simulink library "FriedrichLibrary"  (R2015b)
settings: Solver=ode45  SolverMode=SingleTasking  StartTime=0.0  StopTime=10.0  RelTol=1e-3
values from neighbouring files (symbols this model uses):
  ControlSampleTime = 1/8000    (= 0.000125)    [initTPHardware.m]
  Ts = ControlSampleTime    [Sim_TP3_VSM_init.m]
undefined symbols (not defined in the file or in its folder): init_out
undefined symbols (not defined in the file): CC1, PLL
libraries: FriedrichLibrary x29, simulink x6, powerlib_meascontrol x1
settings Model: Creator=fwelck  LastModifiedBy=fwelck
settings DataIOCC: SaveFormat=Array
settings OptimizationCC: BlockReduction=off  BooleanDataType=off
settings DebuggingCC: SaveWithParameterizedLinksMsg=none  UnderspecifiedInitializationDetection=Classic  MergeDetectMultiDrivingBlocksExec=none  SignalResolutionControl=TryResolveAllWithWarning  StrictBusMsg=Warning
settings HardwareCC: ProdBitPerPointer=32  ProdLargestAtomicFloat=None  ProdIntDivRoundTo=Undefined  ProdEndianess=Unspecified  ProdWordSize=32  ProdHWDeviceType=32-bit Generic  TargetUnknown=on
settings GRTTargetCC: GeneratePreprocessorConditionals=Disable all
settings ConfigComp: CovModelRefEnable=Off  CovSFcnEnable=off

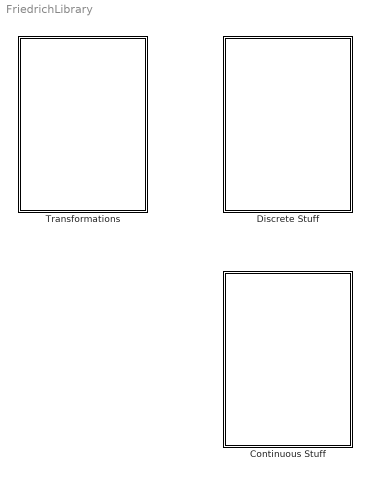
== system FriedrichLibrary ==
  Continuous Stuff : Subsystem
  Discrete Stuff : Subsystem
  Transformations : Subsystem

== system FriedrichLibrary/Continuous Stuff ==
  G.4 First order filter with initial state : Subsystem  mask{T=0.1, init_out=0}
      mask prompts: T "Time constant [s]"; init_out "Initial State"
      mask Display:
      | text(0.5,0.5,'1','HorizontalAlignment','center','VerticalAlignment','Bottom')
      | text(0.5,0.5,['1 + s*' get_param(gcb,'T')],'HorizontalAlignment','center','VerticalAlignment','Top')
      | plot([0.3 0.7],[0.5 0.5])

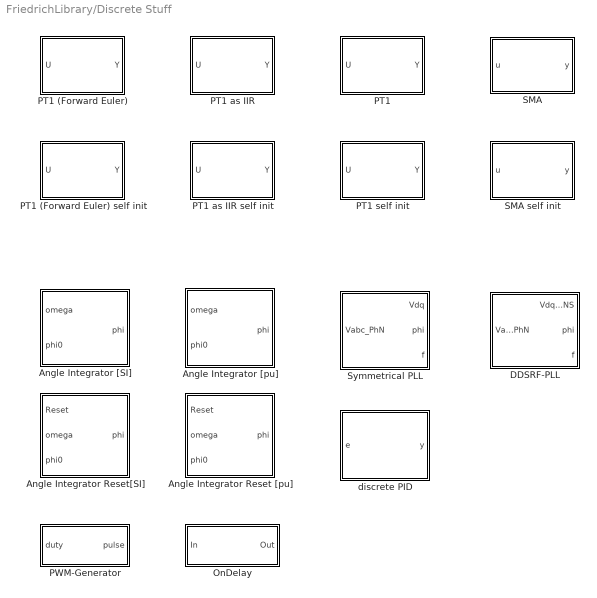
== system FriedrichLibrary/Discrete Stuff ==
  Angle Integrator Reset [pu] : Subsystem  mask{Ts=Ts}
      mask prompts: Ts "SampleTime"
      mask DialogControl DescTextVar Prompt: Discrete Integrator with wrap around at -0.5 and 0.5
  Angle Integrator Reset[SI] : Subsystem  mask{Ts=Ts}
      mask prompts: Ts "SampleTime"
      mask DialogControl DescTextVar Prompt: Discrete Integrator for omega, resetting every 2*pi.
  Angle Integrator [SI] : Subsystem  mask{Ts=Ts}
      mask prompts: Ts "SampleTime"
      mask DialogControl DescTextVar Prompt: Discrete Integrator for omega, resetting every 2*pi.
  Angle Integrator [pu] : Subsystem  mask{Ts=Ts}
      mask prompts: Ts "SampleTime"
      mask DialogControl DescTextVar Prompt: Discrete Integrator with wrap around at -0.5 and 0.5
  DDSRF-PLL : Subsystem  mask{Kp_PLL=PLL.kp, Ki_PLL=PLL.ki, Kd_PLL=0, Tpt1=0.005, Ts=ControlSampleTime}
      mask prompts: Kp_PLL "Proportional Gain PLL"; Ki_PLL "Integral Gain PLL"; Kd_PLL "Differential Gain PLL"; Tpt1 "PT1 Settling Time"; Ts "SampleTime"
      mask DialogControl DescTextVar Prompt: Discrete implementation of a double decoupled sychronous reference frame phase locked loop.
  OnDelay : Subsystem  mask{T_on=2e-6}
      mask prompts: T_on "On Delay Time"
  PT1 : Subsystem  mask{K=1, tau=0.02, Init=0, T=ControlSampleTime}
      mask prompts: K "Gain"; tau "Settling time"; Init "Initial input"; T "Sample time"
      mask DialogControl DescTextVar Prompt: Simple discrete PT1
      mask Display:
      | text(0.5,0.5,get_param(gcb,'K'),'HorizontalAlignment','center','VerticalAlignment','Bottom')
      | text(0.5,0.5,['1 + s*' get_param(gcb,'tau')],'HorizontalAlignment','center','VerticalAlignment','Top')
      | plot([0.3 0.7],[0.5 0.5])
  PT1 self init : Subsystem  mask{K=1, tau=0.02, T=0.001}
      mask prompts: K "Gain"; tau "Settling time"; T "Sample time"
      mask DialogControl DescTextVar Prompt: Simple discrete PT1
      mask Display:
      | text(0.5,0.5,get_param(gcb,'K'),'HorizontalAlignment','center','VerticalAlignment','Bottom')
      | text(0.5,0.5,['1 + s*' get_param(gcb,'tau')],'HorizontalAlignment','center','VerticalAlignment','Top')
      | plot([0.3 0.7],[0.5 0.5])
  PT1 (Forward Euler) : Subsystem  mask{K=1, tau=0.1, Init=0, T=0.001}
      mask prompts: K "Gain"; tau "Settling time [s]"; Init "Initial input"; T "Sample time [s]"
      mask DialogControl DescTextVar Prompt: Forward Euler discretization of a PT1 filter.
      mask Display:
      | text(0.5,0.5,get_param(gcb,'K'),'HorizontalAlignment','center','VerticalAlignment','Bottom')
      | text(0.5,0.5,['1 + s*' get_param(gcb,'tau')],'HorizontalAlignment','center','VerticalAlignment','Top')
      | plot([0.3 0.7],[0.5 0.5])
  PT1 (Forward Euler) self init : Subsystem  mask{K=1, tau=0.1, T=0.001}
      mask prompts: K "Gain"; tau "Settling time [s]"; T "Sample time [s]"
      mask DialogControl DescTextVar Prompt: Forward Euler discretization of a PT1 filter.
      mask Display:
      | text(0.5,0.5,get_param(gcb,'K'),'HorizontalAlignment','center','VerticalAlignment','Bottom')
      | text(0.5,0.5,['1 + s*' get_param(gcb,'tau')],'HorizontalAlignment','center','VerticalAlignment','Top')
      | plot([0.3 0.7],[0.5 0.5])
  PT1 as IIR : Subsystem  mask{K=1, tau=0.02, Init=0, T=ControlSampleTime}
      mask prompts: K "Gain"; tau "Settling time"; Init "Initial input"; T "Sample time"
      mask DialogControl DescTextVar Prompt: IIR form of a PT1 filter
      mask Display:
      | text(0.5,0.5,get_param(gcb,'K'),'HorizontalAlignment','center','VerticalAlignment','Bottom')
      | text(0.5,0.5,['1 + s*' get_param(gcb,'tau')],'HorizontalAlignment','center','VerticalAlignment','Top')
      | plot([0.3 0.7],[0.5 0.5])
  PT1 as IIR self init : Subsystem  mask{K=1, tau=0.02, T=0.001}
      mask prompts: K "Gain"; tau "Settling time"; T "Sample time"
      mask DialogControl DescTextVar Prompt: IIR form of a PT1 filter
      mask Display:
      | text(0.5,0.5,get_param(gcb,'K'),'HorizontalAlignment','center','VerticalAlignment','Bottom')
      | text(0.5,0.5,['1 + s*' get_param(gcb,'tau')],'HorizontalAlignment','center','VerticalAlignment','Top')
      | plot([0.3 0.7],[0.5 0.5])
  PWM-Generator : Subsystem  mask{f_triangle=8000}
      mask prompts: f_triangle "Carrier Frequency"
  SMA : Subsystem  mask{n_samples=3, init_out=0}
      mask prompts: n_samples "Number of samples to average over"; init_out "Initial state"
      mask DialogControl DescTextVar Prompt: Cycle buffer implementation of a simple moving average with initialization. Performs a lot faster than an FIR implementation for averages of 3 samples or more.
  SMA self init : Subsystem  mask{n_samples=3}
      mask prompts: n_samples "Number of samples to average over"
      mask DialogControl DescTextVar Prompt: Cycle buffer implementation of a simple moving average. Performs a lot faster than an FIR implementation for averages of 3 samples or more. Initializes with first input sample.
  Symmetrical PLL : Subsystem  mask{Kp_PLL=CC1.PLL.kp, Ki_PLL=CC1.PLL.ki, Kd_PLL=0, Ts=ControlSampleTime}
      mask prompts: Kp_PLL "Proportional Gain PLL"; Ki_PLL "Integral Gain PLL"; Kd_PLL "Differential Gain PLL"; Ts "SampleTime"
      mask DialogControl DescTextVar Prompt: Discrete implementation of a synchronous reference phase locked loop.
  discrete PID : Subsystem  mask{Kp=1, Ki=2, Kd=3, Ts=ControlSampleTime, x_init=0}
      mask prompts: Kp "Proportional Gain"; Ki "Integral Gain"; Kd "Differential Gain"; Ts "SampleTime"; x_init "Initial Condition"

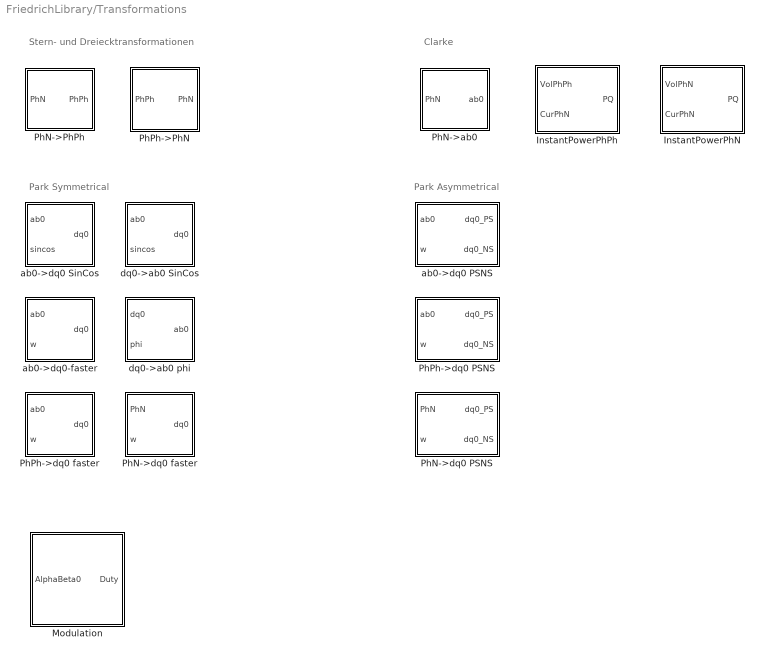
== system FriedrichLibrary/Transformations ==
  note: Park Symmetrical
  note: Park Asymmetrical
  note: Clarke
  note: Stern- und Dreiecktransformationen
  InstantPowerPhN : Subsystem
  InstantPowerPhPh : Subsystem
  Modulation : Subsystem  mask{Method=Sine Modulation, Ts=0}
      mask prompts: Method "Modulation Technique"; Ts "SampleTime"
      mask TypeOptions Method: Standard SpaceVectorModulation | U0N Space Vector Modulation | U7N Space Vector Modulation | Sine Modulation | SineWithThird Modulation
      mask DialogControl DescTextVar Prompt: Performs AlphaBeta0 to ABC conversion via different Modulation Techniques
      mask Display:
      | plot(0,-1,1,1)
      | % Create three 120° shifted sine (3x72)
      | angles = [0:5:360; 120:5:480; 240:5:600]';
      | sine = sind(angles);
      | % Get Maximum and Minimum of all three sine waves
      | Maxi = max(sine,[],2);
      | Mini = min(sine,[],2);
      | % Make them (3x73)
      | Maxi = repmat(Maxi,[1 3]);
      | Mini = repmat(Mini,[1 3]);
      | 
      | switch Method
      |     case 1
      |         plot(angles(:,[1 1 1])/360,sine-(Maxi+Mini)/2);
      |     case 2
      |         plot(angles(:,[1 1 1])/360,sine-Mini-1);
      |     case 3
      |         plot(angles(:,[1 1 1])/360,sine-Maxi+1);
      |     case 4
      |         plot(angles(:,[1 1 1])/360,sine);
      |     case 5
      |         plot(angles(:,[1 1 1])/360,sine-repmat(prod(sine,2)/3*2,[1 3]));
      | end
      | text(0,0,' \alpha\beta0','texmode','on')
      | text(1,0,'duty ','HorizontalAlignment','Right')
  PhN->PhPh : Subsystem
      mask Display:
      | plot([0 1], [0,1])
      | plot([0.1 0.25 0.4 0.25 0.25], [0.5 0.6 0.5 0.6 0.8]) % Stern
      | plot([0.6 0.9 0.75 0.6], [0.2 0.2 0.5 0.2])           % Dreieck
      | text(0.05,1,'PhN','VerticalAlignment','Top')
      | text(1, 0,'PhPh','VerticalAlignment','Bottom','HorizontalAlignment','Right')
  PhN->ab0 : Subsystem
      mask Display:
      | plot([0 1], [0,1])
      | plot([0.1 0.25 0.4 0.25 0.25], [0.5 0.6 0.5 0.6 0.8]) % Stern
      | text(0.05,1,'PhN','VerticalAlignment','Top')
      | text(0.55, 0.3,'\alpha\beta0','texmode','on')
  PhN->dq0 PSNS : Subsystem
      mask Display:
      | plot(0,0,1,1)
      | text(0.05,0.75,'PhN')
      | text(1, 0.75,'dq0_PS','HorizontalAlignment','right')
      | text(1, 0.25,'dq0_NS','HorizontalAlignment','right')
      | text(0.05,0.3,'\phi','texmode','on')
  PhN->dq0 faster : Subsystem
      mask Display:
      | plot([0 1], [0,1])
      | plot([0.1 0.25 0.4 0.25 0.25], [0.5 0.6 0.5 0.6 0.8]) % Stern
      | text(0.05,1,'PhN','VerticalAlignment','Top')
      | text(1, 0.5,'dq0','HorizontalAlignment','right')
      | text(0.05,0.3,'\phi','texmode','on')
  PhPh->PhN : Subsystem
      mask Display:
      | plot([0 1], [0,1])
      | plot([0.6 0.75 0.9 0.75 0.75], [0.2 0.3 0.2 0.3 0.5]) % Stern
      | plot([0.1 0.4 0.25 0.1], [0.5 0.5 0.8 0.5])           % Dreieck
      | text(0.05,1,'PhPh','VerticalAlignment','Top')
      | text(1, 0,'PhN','VerticalAlignment','Bottom','HorizontalAlignment','Right')
  PhPh->dq0 PSNS : Subsystem  mask{Tpt1=0}
      mask prompts: Tpt1 "PT1 Settling Time"
      mask Display:
      | plot(0,0,1,1)
      | text(0.05,0.75,'PhPh')
      | text(1, 0.75,'dq0_PS','HorizontalAlignment','right')
      | text(1, 0.25,'dq0_NS','HorizontalAlignment','right')
      | text(0.05,0.3,'\phi','texmode','on')
  PhPh->dq0 faster : Subsystem
      mask Display:
      | plot([0 1], [0,1])
      | plot([0.1 0.4 0.25 0.1], [0.5 0.5 0.8 0.5])           % Dreieck
      | text(0.05,1,'PhPh','VerticalAlignment','Top')
      | text(1, 0.5,'dq0','HorizontalAlignment','right')
      | text(0.05,0.3,'\phi','texmode','on')
  ab0->dq0 PSNS : Subsystem  mask{T1=0.0045}
      mask prompts: T1 "PT1 Settling Time"
      mask Display:
      | plot(0,0,1,1)
      | text(0.05,0.8,'\alpha\beta0','texmode','on')
      | text(1, 0.75,'dq0_PS','HorizontalAlignment','right')
      | text(1, 0.25,'dq0_NS','HorizontalAlignment','right')
      | text(0.05,0.3,'\phi','texmode','on')
  ab0->dq0 SinCos : Subsystem
      mask Display:
      | plot(0,0,1,1)
      | text(0.05,0.8,'\alpha\beta0','texmode','on')
      | text(1,0.5,'dq0','horizontalalignment','right')
      | text(0.05,0.3,'sincos','texmode','on')
  ab0->dq0-faster : Subsystem
      mask Display:
      | plot([0 1], [0,1])
      | text(0.05,0.8,'\alpha\beta0','texmode','on')
      | text(1, 0.5,'dq0','HorizontalAlignment','right')
      | text(0.05,0.3,'\phi','texmode','on')
  dq0->ab0 SinCos : Subsystem
      mask Display:
      | plot(0,0,1,1)
      | text(0.05,0.8,'dq0')
      | text(1,0.5,'\alpha\beta0','texmode','on','horizontalalignment','right')
      | text(0.05,0.3,'sincos','texmode','on')
  dq0->ab0 phi : Subsystem
      mask Display:
      | plot([0 1], [0,1])
      | text(0.05,0.8,'dq0','texmode','on')
      | text(1, 0.5,'\alpha\beta0','HorizontalAlignment','right','texmode','on')
      | text(0.05,0.3,'\phi','texmode','on')

== system FriedrichLibrary/Continuous Stuff/G.4 First order filter with initial state ==
  x : Inport
  Gain : Gain  Gain=1/T
  Integrator Limited : Integrator  InitialCondition=init_out
  Sum : Sum  Inputs=-+|
  y : Outport
  wires:
  Sum/1 -> Gain/1
  x/1 -> Sum/2
  Gain/1 -> Integrator Limited/1
  Integrator Limited/1 -> Sum/1, y/1

== system FriedrichLibrary/Discrete Stuff/Angle Integrator Reset [pu] ==
  Reset : Inport
  omega : Inport  Port=2
  phi0 : Inport  Port=3
  Bias : Bias  Bias=-1
  Bias1 : Bias  Bias=1
  Delay : Delay  DelayLength=1  InitialConditionSource=Input port  ExternalReset=Rising  SampleTime=Ts
      settings: InputPortMap=u0,r5,p4
  Gain3 : Gain  Gain=Ts
  Sum : Sum  Inputs=|++
  Switch : Switch  Criteria=u2 > Threshold  Threshold=0.5
  Switch1 : Switch  Criteria=u2 > Threshold  Threshold=-0.5
  phi : Outport
  wires:
  phi0/1 -> Delay/3
  Delay/1 -> Sum/2, phi/1
  Switch1/1 -> Delay/1
  Bias1/1 -> Switch1/3
  Switch/1 -> Bias1/1, Switch1/2, Switch1/1
  omega/1 -> Gain3/1
  Gain3/1 -> Sum/1
  Bias/1 -> Switch/1
  Sum/1 -> Switch/3, Switch/2, Bias/1
  Reset/1 -> Delay/2

== system FriedrichLibrary/Discrete Stuff/Angle Integrator Reset[SI] ==
  Reset : Inport
  omega : Inport  Port=2
  phi0 : Inport  Port=3
  Bias : Bias  Bias=-2*pi
  Bias1 : Bias  Bias=2*pi
  Delay : Delay  DelayLength=1  InitialConditionSource=Input port  ExternalReset=Rising  SampleTime=Ts
      settings: InputPortMap=u0,r5,p4
  Gain3 : Gain  Gain=Ts
  Sum : Sum  Inputs=|++
  Switch : Switch  Criteria=u2 > Threshold  Threshold=pi
  Switch1 : Switch  Threshold=-pi
  phi : Outport
  wires:
  Reset/1 -> Delay/2
  phi0/1 -> Delay/3
  omega/1 -> Gain3/1
  Gain3/1 -> Sum/1
  Bias/1 -> Switch/1
  Sum/1 -> Switch/3, Switch/2, Bias/1
  Delay/1 -> phi/1, Sum/2
  Switch/1 -> Switch1/1, Bias1/1, Switch1/2
  Bias1/1 -> Switch1/3
  Switch1/1 -> Delay/1

== system FriedrichLibrary/Discrete Stuff/Angle Integrator [SI] ==
  omega : Inport
  phi0 : Inport  Port=2
  Bias : Bias  Bias=-2*pi
  Bias1 : Bias  Bias=2*pi
  Delay : Delay  DelayLength=1  InitialConditionSource=Input port  SampleTime=Ts
      settings: InputPortMap=u0,p4
  Gain3 : Gain  Gain=Ts
  Sum : Sum  Inputs=|++
  Switch : Switch  Criteria=u2 > Threshold  Threshold=pi
  Switch1 : Switch  Threshold=-pi
  phi : Outport
  wires:
  phi0/1 -> Delay/2
  omega/1 -> Gain3/1
  Gain3/1 -> Sum/1
  Bias/1 -> Switch/1
  Sum/1 -> Switch/3, Switch/2, Bias/1
  Delay/1 -> Sum/2, phi/1
  Switch/1 -> Switch1/1, Bias1/1, Switch1/2
  Bias1/1 -> Switch1/3
  Switch1/1 -> Delay/1

== system FriedrichLibrary/Discrete Stuff/Angle Integrator [pu] ==
  omega : Inport
  phi0 : Inport  Port=2
  Bias : Bias  Bias=-1
  Bias1 : Bias  Bias=1
  Delay : Delay  DelayLength=1  InitialConditionSource=Input port  SampleTime=Ts
      settings: InputPortMap=u0,p4
  Gain3 : Gain  Gain=Ts
  Sum : Sum  Inputs=|++
  Switch : Switch  Criteria=u2 > Threshold  Threshold=0.5
  Switch1 : Switch  Criteria=u2 > Threshold  Threshold=-0.5
  phi : Outport
  wires:
  Sum/1 -> Bias/1, Switch/2, Switch/3
  Bias/1 -> Switch/1
  Gain3/1 -> Sum/1
  omega/1 -> Gain3/1
  Switch/1 -> Switch1/1, Switch1/2, Bias1/1
  Bias1/1 -> Switch1/3
  Switch1/1 -> Delay/1
  Delay/1 -> Sum/2, phi/1
  phi0/1 -> Delay/2

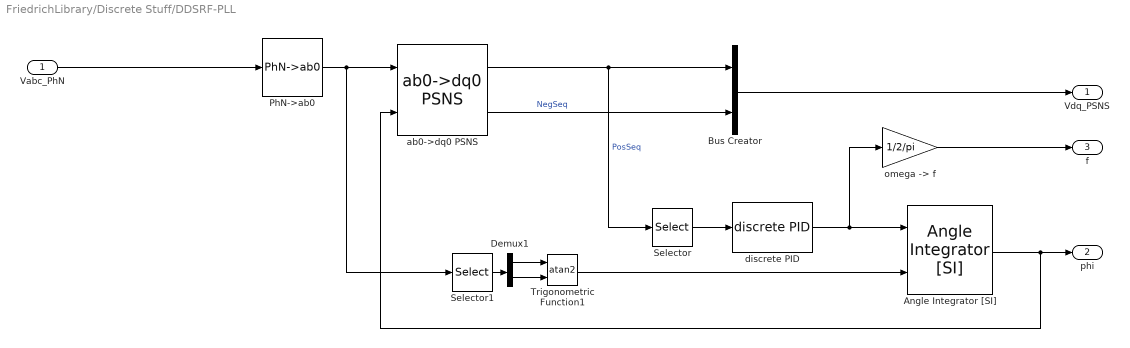
== system FriedrichLibrary/Discrete Stuff/DDSRF-PLL ==
  Vabc_PhN : Inport
  Angle Integrator [SI] : FriedrichLibrary/Discrete Stuff/Angle Integrator [SI]  Ts=Ts
  Bus Creator : BusCreator  Inputs=2
  Demux1 : Demux  Outputs=2
  PhN->ab0 : FriedrichLibrary/Transformations/PhN->ab0  SystemSampleTime=-1
  Selector : Selector  InputPortWidth=3  IndexOptions=Index vector (dialog)  Indices=2  OutputSizes=1
  Selector1 : Selector  InputPortWidth=3  IndexOptions=Index vector (dialog)  Indices=[2 1]  OutputSizes=1
  Trigonometric Function1 : Trigonometry  Operator=atan2
  ab0->dq0 PSNS : FriedrichLibrary/Transformations/ab0->dq0 PSNS  T1=0.0045
  discrete PID : FriedrichLibrary/Discrete Stuff/discrete PID  Kp=Kp_PLL  Ki=Ki_PLL  Kd=Kd_PLL  Ts=Ts  x_init=2*pi*50
  "omega -> f" : Gain  Gain=1/2/pi
  Vdq_PSNS : Outport
  phi : Outport  Port=2
  f : Outport  Port=3
  wires:
  Trigonometric Function1/1 -> Angle Integrator [SI]/2
  PhN->ab0/1 -> Selector1/1, ab0->dq0 PSNS/1
  "omega -> f"/1 -> f/1
  Angle Integrator [SI]/1 -> ab0->dq0 PSNS/2, phi/1
  discrete PID/1 -> "omega -> f"/1, Angle Integrator [SI]/1
  Selector/1 -> discrete PID/1
  ab0->dq0 PSNS/1 -> Selector/1, Bus Creator/1  "PosSeq"
  ab0->dq0 PSNS/2 -> Bus Creator/2  "NegSeq"
  Bus Creator/1 -> Vdq_PSNS/1
  Vabc_PhN/1 -> PhN->ab0/1
  Demux1/2 -> Trigonometric Function1/2
  Selector1/1 -> Demux1/1
  Demux1/1 -> Trigonometric Function1/1

== system FriedrichLibrary/Discrete Stuff/OnDelay ==
  In : Inport
  Logical Operator1 : Logic  AllPortsSameDT=off  OutDataTypeStr=boolean
  Transport Delay : TransportDelay  DelayTime=T_on
  Out : Outport
  wires:
  Transport Delay/1 -> Logical Operator1/2
  In/1 -> Transport Delay/1, Logical Operator1/1
  Logical Operator1/1 -> Out/1

== system FriedrichLibrary/Discrete Stuff/PT1 ==
  U : Inport  SampleTime=T
  Gain : Gain  Gain=T/tau
  Gain1 : Gain  Gain=K
  Sum : Sum  Inputs=|++
  Sum2 : Sum  Inputs=|+-
  Unit Delay1 : UnitDelay  InitialCondition=Init  SampleTime=-1
  Y : Outport
  wires:
  Unit Delay1/1 -> Sum2/2, Sum/2
  Gain/1 -> Sum/1
  U/1 -> Sum2/1
  Sum2/1 -> Gain/1
  Sum/1 -> Gain1/1, Unit Delay1/1
  Gain1/1 -> Y/1

== system FriedrichLibrary/Discrete Stuff/PT1 self init ==
  U : Inport  SampleTime=T
  Constant : Constant  Value=0  VectorParams1D=off  SampleTime=Inf
  Gain : Gain  Gain=T/tau
  Gain1 : Gain  Gain=K
  Initializer : Subsystem
  Sum : Sum  Inputs=|++
  Sum2 : Sum  Inputs=|+-
  Unit Delay2 : Delay  DelayLength=1  InitialConditionSource=Input port
      settings: InputPortMap=u0,p4
  Unit Delay3 : UnitDelay  InitialCondition=1  SampleTime=-1
  Y : Outport
  wires:
  Gain1/1 -> Y/1
  Sum2/1 -> Gain/1
  Gain/1 -> Sum/1
  Sum/1 -> Unit Delay2/1, Gain1/1
  Unit Delay2/1 -> Sum/2, Sum2/2
  U/1 -> Initializer/1(x), Sum2/1
  Constant/1 -> Unit Delay3/1
  Unit Delay3/1 -> Initializer/Enable
  Initializer/1(x0) -> Unit Delay2/2

== system FriedrichLibrary/Discrete Stuff/PT1 (Forward Euler) ==
  U : Inport
  Gain1 : Gain  Gain=K*T/tau
  Gain2 : Gain  Gain=1-T/tau
  Sum : Sum  Inputs=|++
  Unit Delay : UnitDelay  InitialCondition=Init  SampleTime=T
  Unit Delay1 : UnitDelay  InitialCondition=Init*K  SampleTime=T
  Y : Outport
  wires:
  Gain1/1 -> Sum/1
  U/1 -> Unit Delay/1
  Unit Delay/1 -> Gain1/1
  Sum/1 -> Y/1, Unit Delay1/1
  Unit Delay1/1 -> Gain2/1
  Gain2/1 -> Sum/2

== system FriedrichLibrary/Discrete Stuff/PT1 (Forward Euler) self init ==
  U : Inport
  Constant : Constant  Value=0  VectorParams1D=off  SampleTime=Inf
  Gain1 : Gain  Gain=K*T/tau
  Gain2 : Gain  Gain=1-T/tau
  Initializer : Subsystem
  Sum : Sum  Inputs=|++
  Unit Delay : Delay  DelayLength=1  InitialConditionSource=Input port
      settings: InputPortMap=u0,p4
  Unit Delay1 : Delay  DelayLength=1  InitialConditionSource=Input port
      settings: InputPortMap=u0,p4
  Unit Delay2 : UnitDelay  InitialCondition=1  SampleTime=-1
  Y : Outport
  wires:
  Gain2/1 -> Sum/2
  Unit Delay1/1 -> Gain2/1
  Sum/1 -> Unit Delay1/1, Y/1
  Unit Delay/1 -> Gain1/1
  U/1 -> Initializer/1(x), Unit Delay/1
  Gain1/1 -> Sum/1
  Constant/1 -> Unit Delay2/1
  Unit Delay2/1 -> Initializer/Enable
  Initializer/2(x0) -> Unit Delay/2
  Initializer/1(x0*K) -> Unit Delay1/2

== system FriedrichLibrary/Discrete Stuff/PT1 as IIR ==
  U : Inport
  Gain : Gain  Gain=K*T/(T+2*tau)  SampleTime=T
  Gain1 : Gain  Gain=K*T/(T+2*tau)
  Gain2 : Gain  Gain=(T-2*tau)/(T+2*tau)
  Sum : Sum  Inputs=|++
  Sum1 : Sum  Inputs=+|-
  Unit Delay : UnitDelay  InitialCondition=Init  SampleTime=T
  Unit Delay1 : UnitDelay  InitialCondition=Init*K  SampleTime=T
  Y : Outport
  wires:
  U/1 -> Unit Delay/1, Gain/1
  Unit Delay/1 -> Gain1/1
  Gain/1 -> Sum/1
  Sum/1 -> Unit Delay1/1, Y/1
  Unit Delay1/1 -> Gain2/1
  Gain1/1 -> Sum1/1
  Sum1/1 -> Sum/2
  Gain2/1 -> Sum1/2

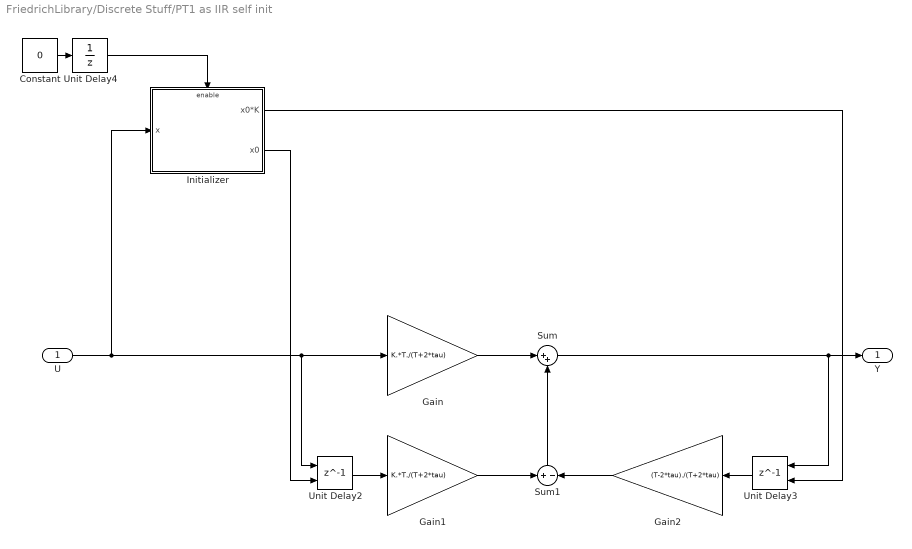
== system FriedrichLibrary/Discrete Stuff/PT1 as IIR self init ==
  U : Inport
  Constant : Constant  Value=0  VectorParams1D=off  SampleTime=Inf
  Gain : Gain  Gain=K.*T./(T+2*tau)  SampleTime=T
  Gain1 : Gain  Gain=K.*T./(T+2*tau)
  Gain2 : Gain  Gain=(T-2*tau)./(T+2*tau)
  Initializer : Subsystem
  Sum : Sum  Inputs=|++
  Sum1 : Sum  Inputs=+|-
  Unit Delay2 : Delay  DelayLength=1  InitialConditionSource=Input port
      settings: InputPortMap=u0,p4
  Unit Delay3 : Delay  DelayLength=1  InitialConditionSource=Input port
      settings: InputPortMap=u0,p4
  Unit Delay4 : UnitDelay  InitialCondition=1  SampleTime=-1
  Y : Outport
  wires:
  Gain2/1 -> Sum1/2
  Sum1/1 -> Sum/2
  Gain1/1 -> Sum1/1
  Unit Delay3/1 -> Gain2/1
  Sum/1 -> Unit Delay3/1, Y/1
  Gain/1 -> Sum/1
  Unit Delay2/1 -> Gain1/1
  U/1 -> Unit Delay2/1, Gain/1, Initializer/1(x)
  Constant/1 -> Unit Delay4/1
  Unit Delay4/1 -> Initializer/Enable
  Initializer/1(x0*K) -> Unit Delay3/2
  Initializer/2(x0) -> Unit Delay2/2

== system FriedrichLibrary/Discrete Stuff/PWM-Generator ==
  duty : Inport
  Data Type Conversion : DataTypeConversion  OutDataTypeStr=double
  Logical Operator : Logic  Operator=NOT  AllPortsSameDT=off  OutDataTypeStr=boolean
  Mux : Mux  Inputs=[3 3]
  Relational Operator : RelationalOperator  OutDataTypeStr=boolean
  Repeating Sequence : simulink/Sources/Repeating Sequence  rep_seq_t=[0 2]  rep_seq_y=[0 2]
  Repeating Sequence1 : simulink/Sources/Repeating Sequence  rep_seq_t=[0 2]  rep_seq_y=[0 2]
  Repeating Sequence2 : simulink/Sources/Repeating Sequence  rep_seq_t=[0 2]  rep_seq_y=[0 2]
  Selector : Selector  InputPortWidth=6  IndexOptions=Index vector (dialog)  Indices=[1 4 2 5 3 6]  OutputSizes=1
  Triangle Generator : powerlib_meascontrol/Pulse & Signal Generators/Triangle Generator  Freq=1e3  Phase=90  Ts=0
  pulse : Outport
  wires:
  duty/1 -> Relational Operator/1
  Repeating Sequence/1 -> Relational Operator/2
  Logical Operator/1 -> Mux/2
  Mux/1 -> Selector/1
  Selector/1 -> Data Type Conversion/1
  Data Type Conversion/1 -> pulse/1
  Relational Operator/1 -> Logical Operator/1, Mux/1

== system FriedrichLibrary/Discrete Stuff/SMA ==
  u : Inport
  Buffer : Delay  DelayLength=n_samples  InitialCondition=repmat([init_out(:)],[1 n_samples])  UseCircularBuffer=on
  Gain : Gain  Gain=1/n_samples
  Integrator : UnitDelay  InitialCondition=init_out*n_samples  SampleTime=-1
  Sum1 : Sum  Inputs=++-
  y : Outport
  wires:
  Gain/1 -> y/1
  Sum1/1 -> Gain/1, Integrator/1
  Buffer/1 -> Sum1/3
  u/1 -> Sum1/2, Buffer/1
  Integrator/1 -> Sum1/1

== system FriedrichLibrary/Discrete Stuff/SMA self init ==
  u : Inport
  Buffer : Delay  DelayLength=n_samples  InitialConditionSource=Input port  InitialCondition=repmat([init_out(:)],[1 n_samples])  UseCircularBuffer=on
      settings: InputPortMap=u0,p4
  Constant : Constant  Value=0  VectorParams1D=off  SampleTime=Inf
  Gain : Gain  Gain=1/n_samples
  Initializer : Subsystem
  Integrator : Delay  DelayLength=1  InitialConditionSource=Input port
      settings: InputPortMap=u0,p4
  Sum : Sum  Inputs=++-
  Unit Delay : UnitDelay  InitialCondition=1  SampleTime=-1
  y : Outport
  wires:
  Integrator/1 -> Sum/1
  Buffer/1 -> Sum/3
  Sum/1 -> Integrator/1, Gain/1
  Gain/1 -> y/1
  Initializer/1(x0 integrator) -> Integrator/2
  Initializer/2(x0 buffer) -> Buffer/2
  Constant/1 -> Unit Delay/1
  Unit Delay/1 -> Initializer/Enable
  u/1 -> Initializer/1(x), Buffer/1, Sum/2

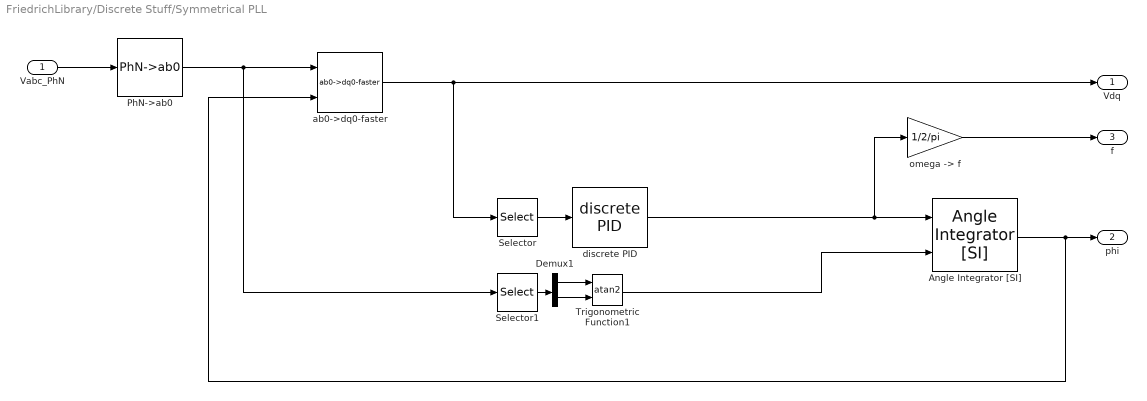
== system FriedrichLibrary/Discrete Stuff/Symmetrical PLL ==
  Vabc_PhN : Inport
  Angle Integrator [SI] : FriedrichLibrary/Discrete Stuff/Angle Integrator [SI]  Ts=Ts
  Demux1 : Demux  Outputs=2
  PhN->ab0 : FriedrichLibrary/Transformations/PhN->ab0  SystemSampleTime=-1
  Selector : Selector  InputPortWidth=3  IndexOptions=Index vector (dialog)  Indices=2  OutputSizes=1
  Selector1 : Selector  InputPortWidth=3  IndexOptions=Index vector (dialog)  Indices=[2 1]  OutputSizes=1
  Trigonometric Function1 : Trigonometry  Operator=atan2
  ab0->dq0-faster : FriedrichLibrary/Transformations/ab0->dq0-faster  SystemSampleTime=-1
  discrete PID : FriedrichLibrary/Discrete Stuff/discrete PID  Kp=Kp_PLL  Ki=Ki_PLL  Kd=Kd_PLL  Ts=Ts  x_init=2*pi*50
  "omega -> f" : Gain  Gain=1/2/pi
  Vdq : Outport
  phi : Outport  Port=2
  f : Outport  Port=3
  wires:
  Trigonometric Function1/1 -> Angle Integrator [SI]/2
  Demux1/2 -> Trigonometric Function1/2
  Demux1/1 -> Trigonometric Function1/1
  Selector1/1 -> Demux1/1
  PhN->ab0/1 -> ab0->dq0-faster/1, Selector1/1
  Vabc_PhN/1 -> PhN->ab0/1
  "omega -> f"/1 -> f/1
  Angle Integrator [SI]/1 -> phi/1, ab0->dq0-faster/2
  discrete PID/1 -> "omega -> f"/1, Angle Integrator [SI]/1
  Selector/1 -> discrete PID/1
  ab0->dq0-faster/1 -> Selector/1, Vdq/1

== system FriedrichLibrary/Discrete Stuff/discrete PID ==
  e : Inport
  Gain : Gain  Gain=Kp
  Gain1 : Gain  Gain=Ki*Ts
  Gain2 : Gain  Gain=Kd/Ts
  Sum1 : Sum  Inputs=+++
  Sum2 : Sum  Inputs=|++
  Sum3 : Sum  Inputs=|-+
  Unit Delay1 : UnitDelay  InitialCondition=x_init  SampleTime=Ts
  Unit Delay2 : UnitDelay  SampleTime=Ts
  y : Outport
  wires:
  Sum3/1 -> Gain2/1
  Gain1/1 -> Sum2/1
  Gain2/1 -> Sum1/3
  Unit Delay1/1 -> Sum2/2
  Gain/1 -> Sum1/1
  Sum1/1 -> y/1
  Unit Delay2/1 -> Sum3/2
  e/1 -> Sum3/1, Unit Delay2/1, Gain1/1, Gain/1
  Sum2/1 -> Unit Delay1/1, Sum1/2

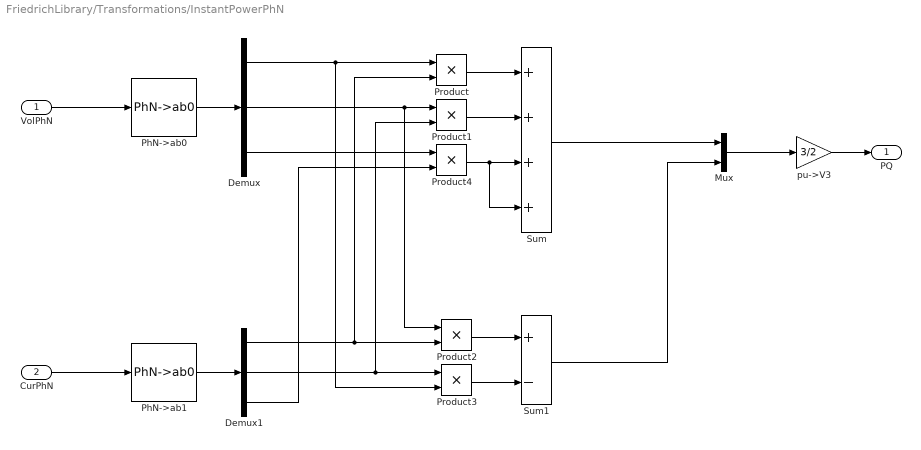
== system FriedrichLibrary/Transformations/InstantPowerPhN ==
  VolPhN : Inport
  CurPhN : Inport  Port=2
  Demux : Demux  Outputs=3
  Demux1 : Demux  Outputs=3
  Mux : Mux  Inputs=2
  PhN->ab0 : FriedrichLibrary/Transformations/PhN->ab0  SystemSampleTime=-1
  PhN->ab1 : FriedrichLibrary/Transformations/PhN->ab0  SystemSampleTime=-1
  Product{,1..4} (5 alike) : Product
  Sum : Sum  Inputs=++++
  Sum1 : Sum  Inputs=+-
  pu->V3 : Gain  Gain=3/2  SaturateOnIntegerOverflow=on  OutDataTypeStr=Inherit: Same as input  ParamDataTypeStr=Inherit: Same as input
  PQ : Outport
  wires:
  pu->V3/1 -> PQ/1
  Mux/1 -> pu->V3/1
  Sum1/1 -> Mux/2
  Sum/1 -> Mux/1
  Product3/1 -> Sum1/2
  Product2/1 -> Sum1/1
  Product1/1 -> Sum/2
  Product/1 -> Sum/1
  Demux1/2 -> Product1/2, Product3/1
  Demux/2 -> Product2/1, Product1/1
  Demux1/1 -> Product/2, Product2/2
  Demux/1 -> Product3/2, Product/1
  PhN->ab1/1 -> Demux1/1
  PhN->ab0/1 -> Demux/1
  CurPhN/1 -> PhN->ab1/1
  VolPhN/1 -> PhN->ab0/1
  Demux/3 -> Product4/1
  Demux1/3 -> Product4/2
  Product4/1 -> Sum/4, Sum/3

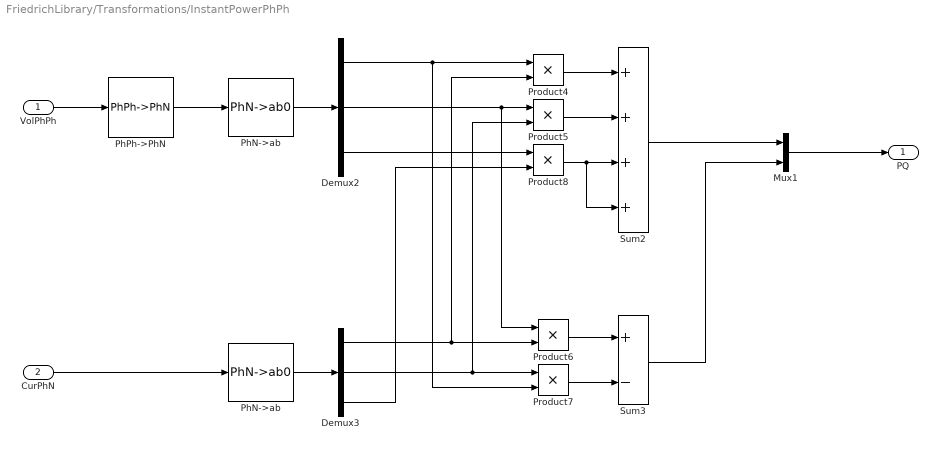
== system FriedrichLibrary/Transformations/InstantPowerPhPh ==
  VolPhPh : Inport
  CurPhN : Inport  Port=2
  Demux2 : Demux  Outputs=3
  Demux3 : Demux  Outputs=3
  Mux1 : Mux  Inputs=2
  PhN->ab : FriedrichLibrary/Transformations/PhN->ab0  SystemSampleTime=-1
  "PhN->ab " : FriedrichLibrary/Transformations/PhN->ab0  SystemSampleTime=-1
  PhPh->PhN : FriedrichLibrary/Transformations/PhPh->PhN  SystemSampleTime=-1
  Product{4..8} (5 alike) : Product
  Sum2 : Sum  Inputs=++++
  Sum3 : Sum  Inputs=+-
  PQ : Outport
  wires:
  VolPhPh/1 -> PhPh->PhN/1
  Mux1/1 -> PQ/1
  Sum3/1 -> Mux1/2
  Sum2/1 -> Mux1/1
  Product7/1 -> Sum3/2
  Product6/1 -> Sum3/1
  Product5/1 -> Sum2/2
  Product4/1 -> Sum2/1
  Demux3/2 -> Product5/2, Product7/1
  Demux2/2 -> Product6/1, Product5/1
  Demux3/1 -> Product4/2, Product6/2
  Demux2/1 -> Product7/2, Product4/1
  "PhN->ab "/1 -> Demux3/1
  PhN->ab/1 -> Demux2/1
  CurPhN/1 -> "PhN->ab "/1
  PhPh->PhN/1 -> PhN->ab/1
  Demux2/3 -> Product8/1
  Demux3/3 -> Product8/2
  Product8/1 -> Sum2/4, Sum2/3

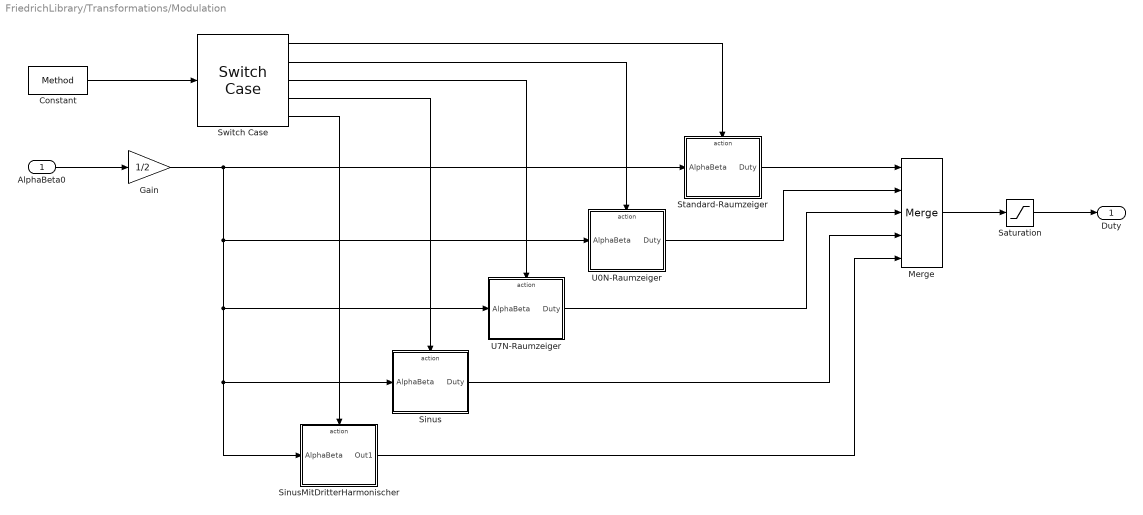
== system FriedrichLibrary/Transformations/Modulation ==
  AlphaBeta0 : Inport
  Constant : Constant  Value=Method  SampleTime=Ts
  Gain : Gain  Gain=1/2
  Merge : Merge  Inputs=5
  Saturation : Saturate  UpperLimit=1  LowerLimit=-1
  Sinus : Subsystem  TreatAsAtomicUnit=on
  SinusMitDritterHarmonischer : Subsystem  TreatAsAtomicUnit=on
  Standard-Raumzeiger : Subsystem  TreatAsAtomicUnit=on
  Switch Case : SwitchCase  CaseConditions={1, 2, 3, 4, 5}  ShowDefaultCase=off
  U0N-Raumzeiger : Subsystem  TreatAsAtomicUnit=on
  U7N-Raumzeiger : Subsystem  TreatAsAtomicUnit=on
  Duty : Outport  SampleTime=Ts
  wires:
  Switch Case/1 -> Standard-Raumzeiger/Action
  Standard-Raumzeiger/1(Duty) -> Merge/1
  Gain/1 -> Standard-Raumzeiger/1(AlphaBeta), Sinus/1(AlphaBeta), SinusMitDritterHarmonischer/1(AlphaBeta), U7N-Raumzeiger/1(AlphaBeta), U0N-Raumzeiger/1(AlphaBeta)
  U0N-Raumzeiger/1(Duty) -> Merge/2
  U7N-Raumzeiger/1(Duty) -> Merge/3
  Sinus/1(Duty) -> Merge/4
  SinusMitDritterHarmonischer/1(Out1) -> Merge/5
  Switch Case/2 -> U0N-Raumzeiger/Action
  Switch Case/3 -> U7N-Raumzeiger/Action
  Switch Case/4 -> Sinus/Action
  Switch Case/5 -> SinusMitDritterHarmonischer/Action
  AlphaBeta0/1 -> Gain/1
  Merge/1 -> Saturation/1
  Saturation/1 -> Duty/1
  Constant/1 -> Switch Case/1

== system FriedrichLibrary/Transformations/PhN->PhPh ==
  PhN : Inport
  SternDreieck : Gain  Gain=[1 -1 0; 0 1 -1; -1 0 1]  Multiplication=Matrix(K*u) (u vector)
  PhPh : Outport
  wires:
  PhN/1 -> SternDreieck/1
  SternDreieck/1 -> PhPh/1

== system FriedrichLibrary/Transformations/PhN->ab0 ==
  PhN : Inport
  AlphaBetaNull Transformation : Gain  Gain="[2/3   -1/3    -1/3;   0   1/sqrt(3) -1/sqrt(3); 1/3 1/3 1/3]"  Multiplication=Matrix(K*u) (u vector)
  ab0 : Outport
  wires:
  PhN/1 -> AlphaBetaNull Transformation/1
  AlphaBetaNull Transformation/1 -> ab0/1

== system FriedrichLibrary/Transformations/PhN->dq0 PSNS ==
  PhN : Inport
  w : Inport  Port=2
  PhN->ab0 : FriedrichLibrary/Transformations/PhN->ab0  SystemSampleTime=-1
  ab0->dq0 PSNS1 : FriedrichLibrary/Transformations/ab0->dq0 PSNS  T1=0.0045
  dq0_PS : Outport
  dq0_NS : Outport  Port=2
  wires:
  w/1 -> ab0->dq0 PSNS1/2
  PhN/1 -> PhN->ab0/1
  PhN->ab0/1 -> ab0->dq0 PSNS1/1
  ab0->dq0 PSNS1/1 -> dq0_PS/1
  ab0->dq0 PSNS1/2 -> dq0_NS/1

== system FriedrichLibrary/Transformations/PhN->dq0 faster ==
  PhN : Inport
  w : Inport  Port=2
  PhN->ab0 : FriedrichLibrary/Transformations/PhN->ab0  SystemSampleTime=-1
  ab0->dq0-faster : FriedrichLibrary/Transformations/ab0->dq0-faster  SystemSampleTime=-1
  dq0 : Outport
  wires:
  ab0->dq0-faster/1 -> dq0/1
  PhN->ab0/1 -> ab0->dq0-faster/1
  PhN/1 -> PhN->ab0/1
  w/1 -> ab0->dq0-faster/2

== system FriedrichLibrary/Transformations/PhPh->PhN ==
  PhPh : Inport
  DreieckStern : Gain  Gain="[1/3   0   -1/3; -1/3   1/3   0; 0  -1/3  1/3 ]"  Multiplication=Matrix(K*u) (u vector)  SaturateOnIntegerOverflow=on  OutDataTypeStr=Inherit: Same as input  ParamDataTypeStr=Inherit: Same as input
  PhN : Outport
  wires:
  PhPh/1 -> DreieckStern/1
  DreieckStern/1 -> PhN/1

== system FriedrichLibrary/Transformations/PhPh->dq0 PSNS ==
  ab0 : Inport
  w : Inport  Port=2
  PhN->ab0 : FriedrichLibrary/Transformations/PhN->ab0  SystemSampleTime=-1
  PhPh->PhN : FriedrichLibrary/Transformations/PhPh->PhN  SystemSampleTime=-1
  ab0->dq0 PSNS : FriedrichLibrary/Transformations/ab0->dq0 PSNS  T1=0.0045
  dq0_PS : Outport
  dq0_NS : Outport  Port=2
  wires:
  ab0->dq0 PSNS/1 -> dq0_PS/1
  PhN->ab0/1 -> ab0->dq0 PSNS/1
  ab0/1 -> PhPh->PhN/1
  PhPh->PhN/1 -> PhN->ab0/1
  w/1 -> ab0->dq0 PSNS/2
  ab0->dq0 PSNS/2 -> dq0_NS/1

== system FriedrichLibrary/Transformations/PhPh->dq0 faster ==
  ab0 : Inport
  w : Inport  Port=2
  PhN->ab0 : FriedrichLibrary/Transformations/PhN->ab0  SystemSampleTime=-1
  PhPh->PhN : FriedrichLibrary/Transformations/PhPh->PhN  SystemSampleTime=-1
  ab0->dq0-faster1 : FriedrichLibrary/Transformations/ab0->dq0-faster  SystemSampleTime=-1
  dq0 : Outport
  wires:
  w/1 -> ab0->dq0-faster1/2
  PhPh->PhN/1 -> PhN->ab0/1
  ab0/1 -> PhPh->PhN/1
  PhN->ab0/1 -> ab0->dq0-faster1/1
  ab0->dq0-faster1/1 -> dq0/1

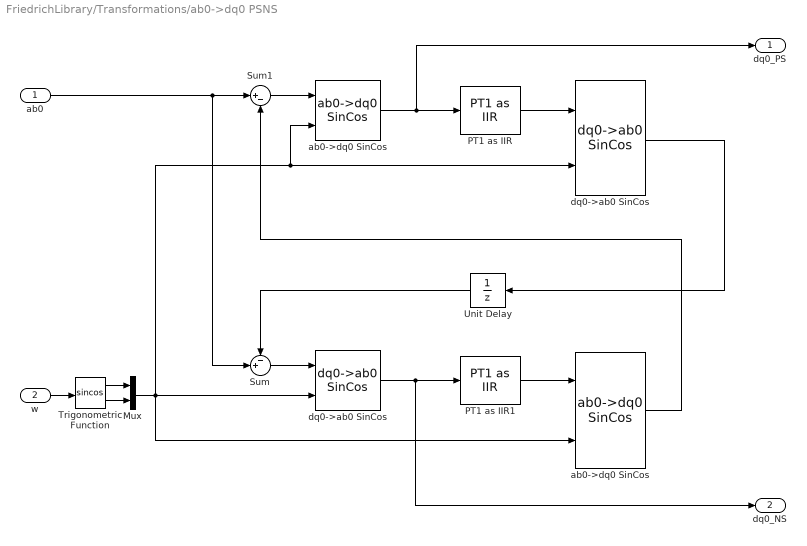
== system FriedrichLibrary/Transformations/ab0->dq0 PSNS ==
  ab0 : Inport
  w : Inport  Port=2
  Mux : Mux  Inputs=2
  PT1 as IIR : FriedrichLibrary/Discrete Stuff/PT1 as IIR  K=1  tau=T1  Init=0  T=ControlSampleTime
  PT1 as IIR1 : FriedrichLibrary/Discrete Stuff/PT1 as IIR  K=1  tau=T1  Init=0  T=ControlSampleTime
  Sum : Sum  Inputs=-+|
  Sum1 : Sum  Inputs=|+-
  Trigonometric Function : Trigonometry  Operator=sincos
  Unit Delay : UnitDelay  SampleTime=-1
  ab0->dq0 SinCos : FriedrichLibrary/Transformations/ab0->dq0 SinCos  SystemSampleTime=-1
  "ab0->dq0 SinCos " : FriedrichLibrary/Transformations/ab0->dq0 SinCos  SystemSampleTime=-1
  dq0->ab0 SinCos : FriedrichLibrary/Transformations/dq0->ab0 SinCos  SystemSampleTime=-1
  "dq0->ab0 SinCos " : FriedrichLibrary/Transformations/dq0->ab0 SinCos  SystemSampleTime=-1
  dq0_PS : Outport
  dq0_NS : Outport  Port=2
  wires:
  ab0/1 -> Sum1/1, Sum/2
  ab0->dq0 SinCos/1 -> PT1 as IIR/1, dq0_PS/1
  dq0->ab0 SinCos/1 -> Unit Delay/1
  Sum/1 -> "dq0->ab0 SinCos "/1
  w/1 -> Trigonometric Function/1
  Trigonometric Function/1 -> Mux/1
  Trigonometric Function/2 -> Mux/2
  Mux/1 -> "dq0->ab0 SinCos "/2, "ab0->dq0 SinCos "/2, ab0->dq0 SinCos/2, dq0->ab0 SinCos/2
  "dq0->ab0 SinCos "/1 -> PT1 as IIR1/1, dq0_NS/1
  "ab0->dq0 SinCos "/1 -> Sum1/2
  Sum1/1 -> ab0->dq0 SinCos/1
  PT1 as IIR/1 -> dq0->ab0 SinCos/1
  PT1 as IIR1/1 -> "ab0->dq0 SinCos "/1
  Unit Delay/1 -> Sum/1

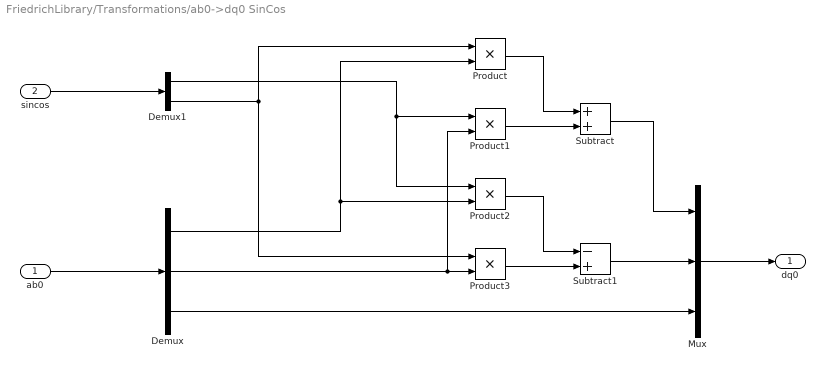
== system FriedrichLibrary/Transformations/ab0->dq0 SinCos ==
  ab0 : Inport
  sincos : Inport  Port=2
  Demux : Demux  Outputs=3
  Demux1 : Demux  Outputs=2
  Mux : Mux  Inputs=3
  Product{,1..3} (4 alike) : Product
  Subtract : Sum
  Subtract1 : Sum  Inputs=-+
  dq0 : Outport
  wires:
  Subtract/1 -> Mux/1
  Subtract1/1 -> Mux/2
  Product3/1 -> Subtract1/2
  Product2/1 -> Subtract1/1
  Product1/1 -> Subtract/2
  Product/1 -> Subtract/1
  Demux1/1 -> Product1/1, Product2/1
  Demux1/2 -> Product/1, Product3/1
  Demux/2 -> Product3/2, Product1/2
  sincos/1 -> Demux1/1
  ab0/1 -> Demux/1
  Demux/1 -> Product/2, Product2/2
  Demux/3 -> Mux/3
  Mux/1 -> dq0/1

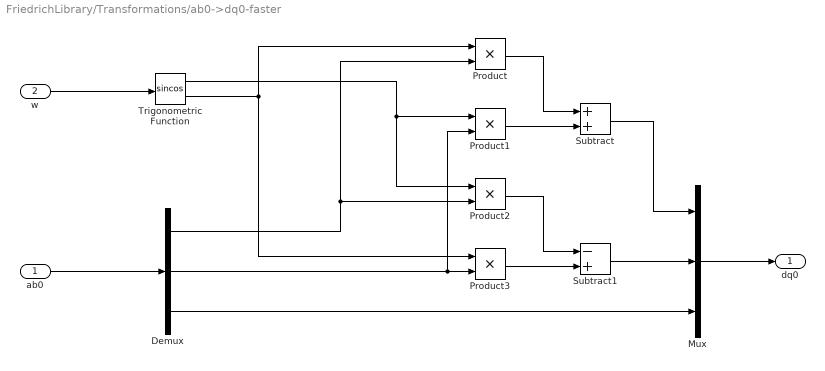
== system FriedrichLibrary/Transformations/ab0->dq0-faster ==
  ab0 : Inport
  w : Inport  Port=2
  Demux : Demux  Outputs=3
  Mux : Mux  Inputs=3
  Product{,1..3} (4 alike) : Product
  Subtract : Sum
  Subtract1 : Sum  Inputs=-+
  Trigonometric Function : Trigonometry  Operator=sincos
  dq0 : Outport
  wires:
  Mux/1 -> dq0/1
  Demux/3 -> Mux/3
  Demux/1 -> Product2/2, Product/2
  ab0/1 -> Demux/1
  w/1 -> Trigonometric Function/1
  Demux/2 -> Product1/2, Product3/2
  Trigonometric Function/2 -> Product/1, Product3/1
  Trigonometric Function/1 -> Product2/1, Product1/1
  Product/1 -> Subtract/1
  Product1/1 -> Subtract/2
  Product2/1 -> Subtract1/1
  Product3/1 -> Subtract1/2
  Subtract1/1 -> Mux/2
  Subtract/1 -> Mux/1

== system FriedrichLibrary/Transformations/dq0->ab0 SinCos ==
  ab0 : Inport
  sincos : Inport  Port=2
  Demux : Demux  Outputs=3
  Demux1 : Demux  Outputs=2
  Mux : Mux  Inputs=3
  Product{,1..3} (4 alike) : Product
  Subtract : Sum  Inputs=+-
  Subtract1 : Sum
  dq0 : Outport
  wires:
  Mux/1 -> dq0/1
  Demux/3 -> Mux/3
  Demux/1 -> Product2/2, Product/2
  ab0/1 -> Demux/1
  sincos/1 -> Demux1/1
  Demux/2 -> Product1/2, Product3/2
  Demux1/2 -> Product3/1, Product/1
  Demux1/1 -> Product2/1, Product1/1
  Product/1 -> Subtract/1
  Product1/1 -> Subtract/2
  Product2/1 -> Subtract1/1
  Product3/1 -> Subtract1/2
  Subtract1/1 -> Mux/2
  Subtract/1 -> Mux/1

== system FriedrichLibrary/Transformations/dq0->ab0 phi ==
  dq0 : Inport
  phi : Inport  Port=2
  Demux : Demux  Outputs=3
  Mux : Mux  Inputs=3
  Product{,1..3} (4 alike) : Product
  Subtract : Sum  Inputs=+-
  Subtract1 : Sum
  Trigonometric Function : Trigonometry  Operator=sincos
  "ab0 " : Outport
  wires:
  phi/1 -> Trigonometric Function/1
  Mux/1 -> "ab0 "/1
  Demux/3 -> Mux/3
  Demux/1 -> Product2/2, Product/2
  dq0/1 -> Demux/1
  Demux/2 -> Product1/2, Product3/2
  Trigonometric Function/2 -> Product/1, Product3/1
  Trigonometric Function/1 -> Product1/1, Product2/1
  Product/1 -> Subtract/1
  Product1/1 -> Subtract/2
  Product2/1 -> Subtract1/1
  Product3/1 -> Subtract1/2
  Subtract1/1 -> Mux/2
  Subtract/1 -> Mux/1

== system FriedrichLibrary/Discrete Stuff/PT1 self init/Initializer ==
  x : Inport
  Enable : EnablePort
  x0 : Outport
  wires:
  x/1 -> x0/1

== system FriedrichLibrary/Discrete Stuff/PT1 (Forward Euler) self init/Initializer ==
  x : Inport
  Enable : EnablePort
  Gain1 : Gain  Gain=K
  x0*K : Outport
  x0 : Outport  Port=2
  wires:
  x/1 -> Gain1/1, x0/1
  Gain1/1 -> x0*K/1

== system FriedrichLibrary/Discrete Stuff/PT1 as IIR self init/Initializer ==
  x : Inport
  Enable : EnablePort
  Gain1 : Gain  Gain=K
  x0*K : Outport
  x0 : Outport  Port=2
  wires:
  x/1 -> Gain1/1, x0/1
  Gain1/1 -> x0*K/1

== system FriedrichLibrary/Discrete Stuff/SMA self init/Initializer ==
  x : Inport
  Enable : EnablePort
  Constant : Constant  Value=ones(1,n_samples)  VectorParams1D=off  SampleTime=Inf
  Gain1 : Gain  Gain=n_samples
  Product : Product  Multiplication=Matrix(*)
  x0 integrator : Outport
  x0 buffer : Outport  Port=2
  wires:
  x/1 -> Gain1/1, Product/1
  Product/1 -> x0 buffer/1
  Constant/1 -> Product/2
  Gain1/1 -> x0 integrator/1

== system FriedrichLibrary/Transformations/Modulation/Sinus ==
  AlphaBeta : Inport
  Action Port : ActionPort
  ab0->duty : Gain  Gain=[2 0 2; -1 sqrt(3) 2; -1 -sqrt(3) 2]  Multiplication=Matrix(K*u) (u vector)
  Duty : Outport
  wires:
  ab0->duty/1 -> Duty/1
  AlphaBeta/1 -> ab0->duty/1

== system FriedrichLibrary/Transformations/Modulation/SinusMitDritterHarmonischer ==
  AlphaBeta : Inport
  Action Port : ActionPort
  Add : Sum  Inputs=+-
  Divide : Product  Inputs=/*
  Gain : Gain  Gain=1/6
  Math Function : Math  Operator=square  SaturateOnIntegerOverflow=on
  Product : Product
  Product of Elements : Product  Inputs=*
  Sqrt : Sqrt  OutputSignalType=real  OutMin=0.001  OutMax=1  SaturateOnIntegerOverflow=on
  Sum of Elements1 : Sum  Inputs=+
  ab0->duty : Gain  Gain=[2 0 2; -1 sqrt(3) 2; -1 -sqrt(3) 2]  Multiplication=Matrix(K*u) (u vector)
  Out1 : Outport
  wires:
  AlphaBeta/1 -> Divide/2, Math Function/1
  Math Function/1 -> Sum of Elements1/1
  Sum of Elements1/1 -> Sqrt/1
  Divide/1 -> ab0->duty/1
  Sqrt/1 -> Divide/1, Product/1  "length"
  ab0->duty/1 -> Add/1, Product of Elements/1
  Product/1 -> Out1/1
  Add/1 -> Product/2
  Product of Elements/1 -> Gain/1
  Gain/1 -> Add/2

== system FriedrichLibrary/Transformations/Modulation/Standard-Raumzeiger ==
  AlphaBeta : Inport
  Action Port : ActionPort
  Merge : Merge  Inputs=4
  Sector 0 and 7 : Subsystem  TreatAsAtomicUnit=on
  Sector 1 and 4 : Subsystem  TreatAsAtomicUnit=on
  Sector 2 and 5 : Subsystem  TreatAsAtomicUnit=on
  Sector 3 and 6 : Subsystem  TreatAsAtomicUnit=on
  SectorFinder : Subsystem
  Switch Case : SwitchCase  CaseConditions={[1,4],[2,5],[3,6],[0 7]}  ShowDefaultCase=off
  Duty : Outport
  wires:
  Switch Case/1 -> Sector 1 and 4/Action
  AlphaBeta/1 -> SectorFinder/1(AlphaBeta), Sector 1 and 4/1(AlphaBeta), Sector 2 and 5/1(AlphaBeta), Sector 3 and 6/1(AlphaBeta)
  Switch Case/2 -> Sector 2 and 5/Action
  Switch Case/3 -> Sector 3 and 6/Action
  Sector 1 and 4/1(Duty) -> Merge/1
  Sector 2 and 5/1(Duty) -> Merge/2
  Sector 3 and 6/1(Duty) -> Merge/3
  Merge/1 -> Duty/1
  Sector 0 and 7/1(Duty) -> Merge/4
  SectorFinder/1(Sector) -> Switch Case/1
  Switch Case/4 -> Sector 0 and 7/Action

== system FriedrichLibrary/Transformations/Modulation/U0N-Raumzeiger ==
  AlphaBeta : Inport
  Action Port : ActionPort
  Merge : Merge  Inputs=4
  Sector 0 and 7 : Subsystem  TreatAsAtomicUnit=on
  Sector 1 and 2 : Subsystem  TreatAsAtomicUnit=on
  Sector 4 and 5 : Subsystem  TreatAsAtomicUnit=on
  Sector 5 and 6 : Subsystem  TreatAsAtomicUnit=on
  SectorFinder : Subsystem
  Switch Case : SwitchCase  CaseConditions={[1,2],[3,4],[5,6],[0 7]}  ShowDefaultCase=off
  Duty : Outport
  wires:
  Switch Case/4 -> Sector 0 and 7/Action
  Sector 0 and 7/1(Duty) -> Merge/4
  Merge/1 -> Duty/1
  Sector 5 and 6/1(Duty) -> Merge/3
  Sector 4 and 5/1(Duty) -> Merge/2
  Sector 1 and 2/1(Duty) -> Merge/1
  Switch Case/3 -> Sector 5 and 6/Action
  Switch Case/2 -> Sector 4 and 5/Action
  AlphaBeta/1 -> Sector 5 and 6/1(AlphaBeta), Sector 4 and 5/1(AlphaBeta), Sector 1 and 2/1(AlphaBeta), SectorFinder/1(AlphaBeta)
  Switch Case/1 -> Sector 1 and 2/Action
  SectorFinder/1(Sector) -> Switch Case/1

== system FriedrichLibrary/Transformations/Modulation/U7N-Raumzeiger ==
  AlphaBeta : Inport
  Action Port : ActionPort
  Merge : Merge  Inputs=4
  Sector 0 and 7 : Subsystem  TreatAsAtomicUnit=on
  Sector 2 and 3 : Subsystem  TreatAsAtomicUnit=on
  Sector 4 and 5 : Subsystem  TreatAsAtomicUnit=on
  Sector 6 and 1 : Subsystem  TreatAsAtomicUnit=on
  SectorFinder : Subsystem
  Switch Case : SwitchCase  CaseConditions={[2,3],[4,5],[6,1],[0 7]}  ShowDefaultCase=off
  Duty : Outport
  wires:
  Switch Case/1 -> Sector 2 and 3/Action
  AlphaBeta/1 -> Sector 2 and 3/1(AlphaBeta), Sector 4 and 5/1(AlphaBeta), Sector 6 and 1/1(AlphaBeta), SectorFinder/1(AlphaBeta)
  Switch Case/2 -> Sector 4 and 5/Action
  Switch Case/3 -> Sector 6 and 1/Action
  Sector 2 and 3/1(Duty) -> Merge/1
  Sector 4 and 5/1(Duty) -> Merge/2
  Sector 6 and 1/1(Duty) -> Merge/3
  Merge/1 -> Duty/1
  Sector 0 and 7/1(Duty) -> Merge/4
  Switch Case/4 -> Sector 0 and 7/Action
  SectorFinder/1(Sector) -> Switch Case/1

== system FriedrichLibrary/Transformations/Modulation/Standard-Raumzeiger/Sector 0 and 7 ==
  Action Port : ActionPort
  Constant : Constant  Value=[1 1 1]
  Duty : Outport  InitialOutput=[0 0 0]
  wires:
  Constant/1 -> Duty/1

== system FriedrichLibrary/Transformations/Modulation/Standard-Raumzeiger/Sector 1 and 4 ==
  AlphaBeta : Inport
  Action Port : ActionPort
  "ab0 -> duty" : Gain  Gain="[3/2   sqrt(3)/2   2; -3/2   3*sqrt(3)/2   2; -3/2  -sqrt(3)/2  2]"  Multiplication=Matrix(K*u) (u vector)  SaturateOnIntegerOverflow=on  OutDataTypeStr=Inherit: Same as input  ParamDataTypeStr=Inherit: Same as input
  Duty : Outport
  wires:
  AlphaBeta/1 -> "ab0 -> duty"/1
  "ab0 -> duty"/1 -> Duty/1

== system FriedrichLibrary/Transformations/Modulation/Standard-Raumzeiger/Sector 2 and 5 ==
  AlphaBeta : Inport
  Action Port : ActionPort
  "ab0 -> duty" : Gain  Gain="[3   0   2; 0   sqrt(3)   2; 0  -sqrt(3)  2]"  Multiplication=Matrix(K*u) (u vector)  SaturateOnIntegerOverflow=on  OutDataTypeStr=Inherit: Same as input  ParamDataTypeStr=Inherit: Same as input
  Duty : Outport
  wires:
  "ab0 -> duty"/1 -> Duty/1
  AlphaBeta/1 -> "ab0 -> duty"/1

== system FriedrichLibrary/Transformations/Modulation/Standard-Raumzeiger/Sector 3 and 6 ==
  AlphaBeta : Inport
  Action Port : ActionPort
  "ab0 -> duty" : Gain  Gain="[3/2   -sqrt(3)/2   2; -3/2   sqrt(3)/2   2; -3/2  -3*sqrt(3)/2  2]"  Multiplication=Matrix(K*u) (u vector)  SaturateOnIntegerOverflow=on  OutDataTypeStr=Inherit: Same as input  ParamDataTypeStr=Inherit: Same as input
  Duty : Outport
  wires:
  AlphaBeta/1 -> "ab0 -> duty"/1
  "ab0 -> duty"/1 -> Duty/1

== system FriedrichLibrary/Transformations/Modulation/Standard-Raumzeiger/SectorFinder ==
  AlphaBeta : Inport
  1-D Lookup Table1 : Lookup_n-D  NumberOfTableDimensions=1  BreakpointsForDimension1=[0 1 2 3 4 5 6 7]  IndexSearchMethod=Evenly spaced points  Table=[1 2 0 3 6 7 5 4]  InterpMethod=Nearest  InternalRulePriority=Speed  RndMeth=Simplest  InputSameDT=on
  Compare To Zero2 : simulink/Logic and Bit Operations/Compare To Zero  relop=<=  OutDataTypeStr=boolean
  Gain3 : Gain  Gain=[0 1 0;sqrt(3) 1 0;sqrt(3) -1 0]  Multiplication=Matrix(K*u)
  Gain4 : Gain  Gain=[4 2 1]  Multiplication=Matrix(K*u)  ParamDataTypeStr=double
  Sector : Outport
  wires:
  1-D Lookup Table1/1 -> Sector/1
  Gain4/1 -> 1-D Lookup Table1/1
  Compare To Zero2/1 -> Gain4/1
  Gain3/1 -> Compare To Zero2/1
  AlphaBeta/1 -> Gain3/1

== system FriedrichLibrary/Transformations/Modulation/U0N-Raumzeiger/Sector 0 and 7 ==
  Action Port : ActionPort
  Constant : Constant  Value=[-1 -1 -1]
  Duty : Outport  InitialOutput=[-1 -1 -1]
  wires:
  Constant/1 -> Duty/1

== system FriedrichLibrary/Transformations/Modulation/U0N-Raumzeiger/Sector 1 and 2 ==
  AlphaBeta : Inport
  Action Port : ActionPort
  Bias : Bias  Bias=[-1 -1 -1]
  "ab0 -> duty" : Gain  Gain="[3   sqrt(3)   1; 0   2*sqrt(3)   1; 0  0  0 ]"  Multiplication=Matrix(K*u) (u vector)  SaturateOnIntegerOverflow=on  OutDataTypeStr=Inherit: Same as input  ParamDataTypeStr=Inherit: Same as input
  Duty : Outport
  wires:
  "ab0 -> duty"/1 -> Bias/1
  AlphaBeta/1 -> "ab0 -> duty"/1
  Bias/1 -> Duty/1

== system FriedrichLibrary/Transformations/Modulation/U0N-Raumzeiger/Sector 4 and 5 ==
  AlphaBeta : Inport
  Action Port : ActionPort
  Bias : Bias  Bias=[-1 -1 -1]
  "ab0 -> duty" : Gain  Gain="[0   0   0; -3   sqrt(3)   1; -3  -sqrt(3)  1]"  Multiplication=Matrix(K*u) (u vector)  SaturateOnIntegerOverflow=on  OutDataTypeStr=Inherit: Same as input  ParamDataTypeStr=Inherit: Same as input
  Duty : Outport
  wires:
  Bias/1 -> Duty/1
  AlphaBeta/1 -> "ab0 -> duty"/1
  "ab0 -> duty"/1 -> Bias/1

== system FriedrichLibrary/Transformations/Modulation/U0N-Raumzeiger/Sector 5 and 6 ==
  AlphaBeta : Inport
  Action Port : ActionPort
  Bias : Bias  Bias=[-1 -1 -1]
  "ab0 -> duty" : Gain  Gain="[3   -sqrt(3)   1; 0   0   0; 0  -2*sqrt(3)  1]"  Multiplication=Matrix(K*u) (u vector)  SaturateOnIntegerOverflow=on  OutDataTypeStr=Inherit: Same as input  ParamDataTypeStr=Inherit: Same as input
  Duty : Outport
  wires:
  "ab0 -> duty"/1 -> Bias/1
  AlphaBeta/1 -> "ab0 -> duty"/1
  Bias/1 -> Duty/1

== system FriedrichLibrary/Transformations/Modulation/U0N-Raumzeiger/SectorFinder ==
  AlphaBeta : Inport
  1-D Lookup Table1 : Lookup_n-D  NumberOfTableDimensions=1  BreakpointsForDimension1=[0 1 2 3 4 5 6 7]  IndexSearchMethod=Evenly spaced points  Table=[1 2 0 3 6 7 5 4]  InterpMethod=Nearest  InternalRulePriority=Speed  RndMeth=Simplest  InputSameDT=on
  Compare To Zero2 : simulink/Logic and Bit Operations/Compare To Zero  relop=<=  OutDataTypeStr=boolean
  Gain3 : Gain  Gain=[0 1 0;sqrt(3) 1 0;sqrt(3) -1 0]  Multiplication=Matrix(K*u)
  Gain4 : Gain  Gain=[4 2 1]  Multiplication=Matrix(K*u)  ParamDataTypeStr=double
  Sector : Outport
  wires:
  1-D Lookup Table1/1 -> Sector/1
  Gain4/1 -> 1-D Lookup Table1/1
  Compare To Zero2/1 -> Gain4/1
  Gain3/1 -> Compare To Zero2/1
  AlphaBeta/1 -> Gain3/1

== system FriedrichLibrary/Transformations/Modulation/U7N-Raumzeiger/Sector 0 and 7 ==
  Action Port : ActionPort
  Constant : Constant  Value=[1 1 1]
  Duty : Outport  InitialOutput=[1 1 1]
  wires:
  Constant/1 -> Duty/1

== system FriedrichLibrary/Transformations/Modulation/U7N-Raumzeiger/Sector 2 and 3 ==
  AlphaBeta : Inport
  Action Port : ActionPort
  Bias : Bias  Bias=1
  "ab0 -> duty" : Gain  Gain="[3   -sqrt(3)   1; 0   0   0; 0  -2*sqrt(3)  1]"  Multiplication=Matrix(K*u) (u vector)  SaturateOnIntegerOverflow=on  OutDataTypeStr=Inherit: Same as input  ParamDataTypeStr=Inherit: Same as input
  Duty : Outport
  wires:
  Bias/1 -> Duty/1
  AlphaBeta/1 -> "ab0 -> duty"/1
  "ab0 -> duty"/1 -> Bias/1

== system FriedrichLibrary/Transformations/Modulation/U7N-Raumzeiger/Sector 4 and 5 ==
  AlphaBeta : Inport
  Action Port : ActionPort
  Bias : Bias  Bias=1
  "ab0 -> duty" : Gain  Gain="[3  sqrt(3)  1; 0  2*sqrt(3)   1; 0   0   0]"  Multiplication=Matrix(K*u) (u vector)  SaturateOnIntegerOverflow=on  OutDataTypeStr=Inherit: Same as input  ParamDataTypeStr=Inherit: Same as input
  Duty : Outport
  wires:
  "ab0 -> duty"/1 -> Bias/1
  AlphaBeta/1 -> "ab0 -> duty"/1
  Bias/1 -> Duty/1

== system FriedrichLibrary/Transformations/Modulation/U7N-Raumzeiger/Sector 6 and 1 ==
  AlphaBeta : Inport
  Action Port : ActionPort
  Bias : Bias  Bias=1
  "ab0 -> duty" : Gain  Gain="[0   0   0; -3   sqrt(3)   1; -3   -sqrt(3)   1]"  Multiplication=Matrix(K*u) (u vector)  SaturateOnIntegerOverflow=on  OutDataTypeStr=Inherit: Same as input  ParamDataTypeStr=Inherit: Same as input
  Duty : Outport
  wires:
  Bias/1 -> Duty/1
  AlphaBeta/1 -> "ab0 -> duty"/1
  "ab0 -> duty"/1 -> Bias/1

== system FriedrichLibrary/Transformations/Modulation/U7N-Raumzeiger/SectorFinder ==
  AlphaBeta : Inport
  1-D Lookup Table1 : Lookup_n-D  NumberOfTableDimensions=1  BreakpointsForDimension1=[0 1 2 3 4 5 6 7]  IndexSearchMethod=Evenly spaced points  Table=[1 2 0 3 6 7 5 4]  InterpMethod=Nearest  InternalRulePriority=Speed  RndMeth=Simplest  InputSameDT=on
  Compare To Zero2 : simulink/Logic and Bit Operations/Compare To Zero  relop=<=  OutDataTypeStr=boolean
  Gain3 : Gain  Gain=[0 1 0;sqrt(3) 1 0;sqrt(3) -1 0]  Multiplication=Matrix(K*u)
  Gain4 : Gain  Gain=[4 2 1]  Multiplication=Matrix(K*u)  ParamDataTypeStr=double
  Sector : Outport
  wires:
  1-D Lookup Table1/1 -> Sector/1
  Gain4/1 -> 1-D Lookup Table1/1
  Compare To Zero2/1 -> Gain4/1
  Gain3/1 -> Compare To Zero2/1
  AlphaBeta/1 -> Gain3/1
